simulink model "ukf_cfg1"  (R2013b)
settings: Solver=FixedStepDiscrete  StartTime=0.0  StopTime=59  FixedStep=0.0001  RelTol=1e-3
InitFcn:
  | %p = pwd;
  | %idx = strfind(p,'\')
  | %addpath(p(1:max(idx)-1))
  | dT=0.0001
settings Model: PauseTimes=93.4  SnapshotBufferSize=5  SnapshotInterval=5  Creator=igeorgie  LastModifiedBy=igeorgie

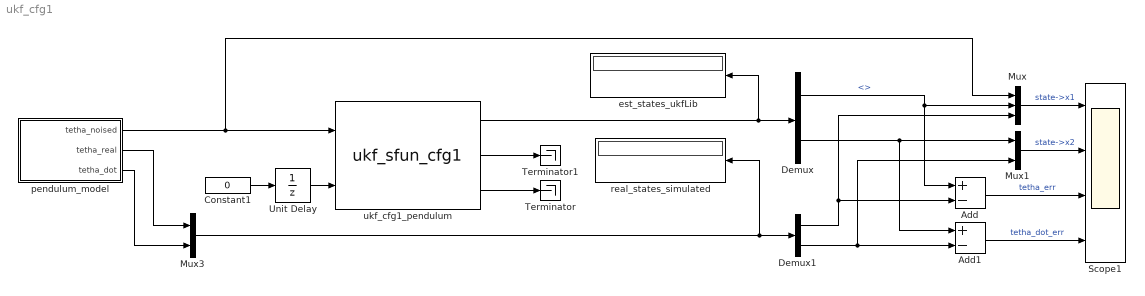
== system ukf_cfg1 ==
  Add : Sum  Inputs=+-
  Add1 : Sum  Inputs=+-
  Constant1 : Constant  Value=0  OutDataTypeStr=double  SampleTime=0.1
  Demux : Demux  Outputs=2
  Demux1 : Demux  Outputs=2
  Mux : Mux  Inputs=3
  Mux1 : Mux  Inputs=2
  Mux3 : Mux  Inputs=2
  Scope1 : Scope  NumInputPorts=4
      settings: TickLabels=on  YMin=-5~-5~-5~-5  YMax=5~5~5~5
  Terminator : Terminator
  Terminator1 : Terminator
  Unit Delay : UnitDelay  InitialCondition=1  SampleTime=0.1
  est_states_ukfLib : Display
  pendulum_model : Subsystem
  real_states_simulated : Display
  ukf_cfg1_pendulum : S-Function  InitFcn=try, set_param(gcb,'FunctionName','ukf_sfun_cfg1'), end  FunctionName=ukf_sfun_cfg1  SFunctionModules=ukf_sfun_cfg1_wrapper ukfLib mtxLib ukfCfg1  EnableBusSupport=off  mask(S-Function Builder){}
      mask help: Simulink:masks:SFunctionBuilder_MD
      mask init:
      | val = [[.9  0.75 0.75 1 1 .9 .9 1]',[1 1 0.75 0.75 .9 .9 1 .9]'];try , sys = get_param(gcb,'SfunBuilderFcnName');if isempty(sys), sys = get_param(gcb,'FunctionName'); end,catch, sys = get_param(gcb,'FunctionName'); end
      settings: CopyFcn=set_param(gcbh,'LinkStatus','none')  PreSaveFcn=try, set_param(gcb,'FunctionName','ukf_sfun_cfg1'), end  OpenFcn=sfunctionwizard(gcbh)
      mask Display: plot(val(:,1),val(:,2)),disp(sys), port_label('input',1,'meas'), port_label('input',2,'Init'), port_label('output',1,'states'), port_label('output',2,'y_mean'), port_label('output',3,'kalman')
  wires:
  Unit Delay/1 -> ukf_cfg1_pendulum/2
  Constant1/1 -> Unit Delay/1
  ukf_cfg1_pendulum/1 -> Demux/1, est_states_ukfLib/1
  ukf_cfg1_pendulum/3 -> Terminator/1
  Demux/1 -> Mux/2, Add/1  "<>"
  Demux1/1 -> Mux/3, Add/2
  Demux/2 -> Add1/1, Mux1/1
  Demux1/2 -> Add1/2, Mux1/2
  Mux/1 -> Scope1/1  "state->x1"
  Mux1/1 -> Scope1/2  "state->x2"
  Mux3/1 -> real_states_simulated/1, Demux1/1
  pendulum_model/1(tetha_noised) -> Mux/1, ukf_cfg1_pendulum/1
  ukf_cfg1_pendulum/2 -> Terminator1/1
  pendulum_model/3(tetha_dot) -> Mux3/2
  Add/1 -> Scope1/3  "tetha_err"
  Add1/1 -> Scope1/4  "tetha_dot_err"
  pendulum_model/2(tetha_real) -> Mux3/1

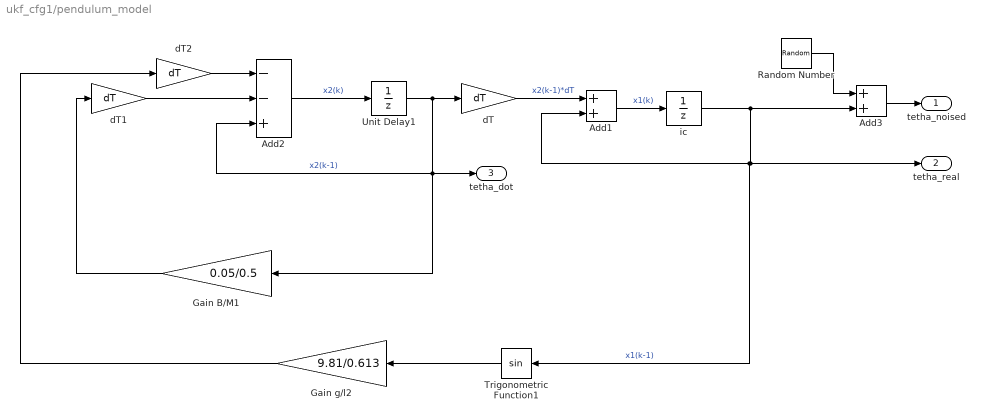
== system ukf_cfg1/pendulum_model ==
  Add1 : Sum
  Add2 : Sum  Inputs=--+
  Add3 : Sum
  Gain B/M1 : Gain  Gain=0.05/0.5
  Gain g/l2 : Gain  Gain=9.81/0.613
  Random Number : RandomNumber  Variance=pi/1000  SampleTime=0.0001
  Trigonometric Function1 : Trigonometry
  Unit Delay1 : UnitDelay  SampleTime=-1
  dT : Gain  Gain=dT
  dT1 : Gain  Gain=dT
  dT2 : Gain  Gain=dT
  ic : UnitDelay  InitialCondition=-pi/4  SampleTime=-1
  tetha_noised : Outport
  tetha_real : Outport  Port=2
  tetha_dot : Outport  Port=3
  wires:
  Gain g/l2/1 -> dT2/1
  Unit Delay1/1 -> tetha_dot/1, Gain B/M1/1, Add2/3, dT/1  "x2(k-1)"
  Trigonometric Function1/1 -> Gain g/l2/1
  Add1/1 -> ic/1  "x1(k)"
  Gain B/M1/1 -> dT1/1
  dT2/1 -> Add2/1
  ic/1 -> Add3/2, Trigonometric Function1/1, Add1/2, tetha_real/1  "x1(k-1)"
  dT/1 -> Add1/1  "x2(k-1)*dT"
  dT1/1 -> Add2/2
  Add2/1 -> Unit Delay1/1  "x2(k)"
  Random Number/1 -> Add3/1
  Add3/1 -> tetha_noised/1
